simulink model "Moj_model"  (R2020a)
settings: Solver=VariableStepAuto  StartTime=0.0  StopTime=0.1  RelTol=1e-3
values from neighbouring files (symbols this model uses):
  g = 9.81    [Dane_moj_model.m]
  h = 0.0012    [Dane_moj_model.m]
  i_e = x_e*sqrt(g/h)    [Dane_moj_model.m]
  L = 0.150    (= 0.15)    [Dane_moj_model.m]
  q = 0    [Dane_moj_model.m]
  R = 5    [Dane_moj_model.m]
  v_e = 0    [Dane_moj_model.m]
  x_e = 0.010    (= 0.01)    [Dane_moj_model.m]
settings Model: Creator=Student  LastModifiedBy=Michał
settings DataIOCC: ReturnWorkspaceOutputs=off
settings DebuggingCC: ArithmeticOperatorsInVariantConditions=warning
settings SFSimCC: CustomCodeUndefinedFunction=UseInterfaceOnly

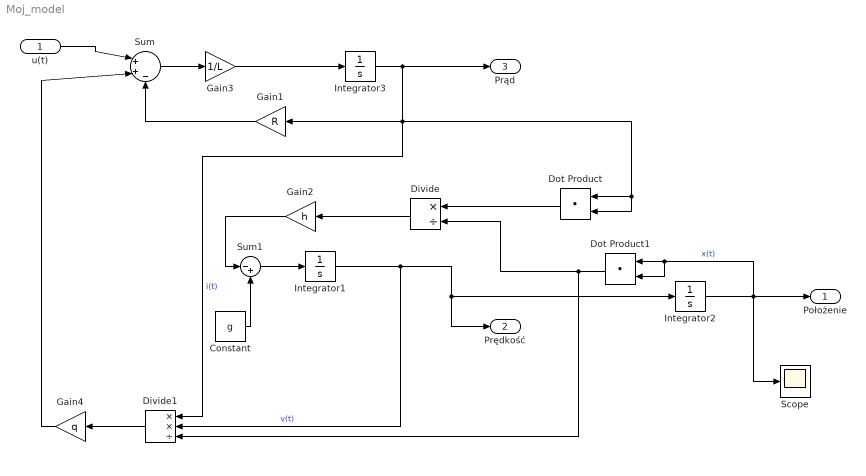
== system Moj_model ==
  u(t) : Inport
  Constant : Constant  Value=g
  Divide : Product  Inputs=*/
  Divide1 : Product  Inputs=**/
  Dot Product : DotProduct  InputSameDT=on  OutDataTypeStr=Inherit: Inherit via internal rule
  Dot Product1 : DotProduct  InputSameDT=on  OutDataTypeStr=Inherit: Inherit via internal rule
  Gain1 : Gain  Gain=R
  Gain2 : Gain  Gain=h
  Gain3 : Gain  Gain=1/L
  Gain4 : Gain  Gain=q
  Integrator1 : Integrator  InitialCondition=v_e
  Integrator2 : Integrator  InitialCondition=x_e
  Integrator3 : Integrator  InitialCondition=i_e
  Scope : Scope
  Sum : Sum  Inputs=|++-
  Sum1 : Sum  Inputs=|-+
  " Położenie " : Outport  VectorParamsAs1DForOutWhenUnconnected=off
  "Prędkość " : Outport  Port=2  VectorParamsAs1DForOutWhenUnconnected=off
  Prąd : Outport  Port=3  VectorParamsAs1DForOutWhenUnconnected=off
  wires:
  Gain4/1 -> Sum/2
  Dot Product/1 -> Divide/1
  Integrator3/1 -> Prąd/1, Gain1/1, Divide1/1, Dot Product/2, Dot Product/1  "i(t)"
  Gain1/1 -> Sum/3
  Constant/1 -> Sum1/2
  Dot Product1/1 -> Divide1/3, Divide/2
  Sum1/1 -> Integrator1/1
  Sum/1 -> Gain3/1
  Gain3/1 -> Integrator3/1
  Divide/1 -> Gain2/1
  Integrator2/1 -> " Położenie "/1, Scope/1, Dot Product1/1, Dot Product1/2  "x(t)"
  Gain2/1 -> Sum1/1
  Integrator1/1 -> "Prędkość "/1, Integrator2/1, Divide1/2  "v(t)"
  Divide1/1 -> Gain4/1
  u(t)/1 -> Sum/1
